simulink model "ejemplo_simulink_completo_vel_lineal_2"  (R2018a)
settings: Solver=FixedStepDiscrete  StartTime=0.0  StopTime=inf  FixedStep=0.001  RelTol=1e-3  EnableMultiTasking=on
libraries: vrlib x1, aerolibanimutils x1
settings Model: Creator=PC  LastModifiedBy=emder
settings OptimizationCC: LifeSpan=inf
settings DebuggingCC: SFUnexpectedBacktrackingDiag=warning  SFNoUnconditionalDefaultTransitionDiag=warning  SFExecutionAtInitializationDiag=none
settings CodeAppCC: StateflowObjectComments=on
settings GRTTargetCC: TargetLangStandard=C89/C90 (ANSI)  GeneratePreprocessorConditionals=Disable all
settings ConfigComp: CovMetricSettings=dw  CovHtmlReporting=on  CovSaveCumulativeToWorkspaceVar=on  CovSaveSingleToWorkspaceVar=on  CovExternalEMLEnable=off

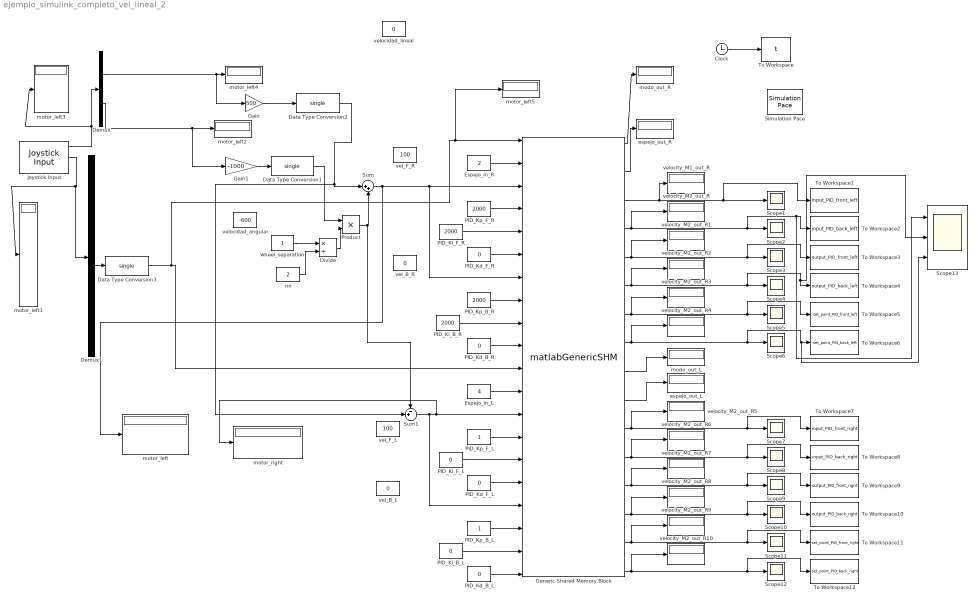
== system ejemplo_simulink_completo_vel_lineal_2 ==
  Clock : Clock
  Data Type Conversion1 : DataTypeConversion  OutDataTypeStr=single
  Data Type Conversion2 : DataTypeConversion  OutDataTypeStr=single
  Data Type Conversion3 : DataTypeConversion  OutDataTypeStr=single
  Demux : Demux  Outputs=5
  Demux1 : Demux  Outputs=10
  Divide : Product  Inputs=*/
  Espejo_in_L : Constant  Value=4  OutDataTypeStr=single
  Espejo_in_R : Constant  Value=2  OutDataTypeStr=single
  Gain : Gain  Gain=500
  Gain1 : Gain  Gain=-1000
  Generic Shared Memory Block : S-Function  FunctionName=matlabGenericSHM  Parameters=nombre,dispositivo,vecE,vecS,tipoE,tipoS,ts  SFunctionDeploymentMode=off  EnableBusSupport=off  mask(Generic Share Memory block V2.0){nombre='ARDUINO', dispositivo=1, vecE=[1 1 1 1 1 1 1 1 1 1 1 1 1 1 1 1 1 1 1 1], vecS=[1 1 1 1 1 1 1 1 1 1 1 1 1 1 1 1], tipoE=['f' 'f' 'f' 'f' 'f' 'f' 'f' 'f' 'f' 'f' 'f' 'f' 'f' 'f' 'f' 'f' 'f' 'f' 'f' 'f'], tipoS=['f' 'f' 'f' 'f' 'f' 'f' 'f' 'f' 'f' 'f' 'f' 'f' 'f' 'f' 'f' 'f'], ts=-1}
      mask prompts: nombre "Share Memory base name"; dispositivo "Device Number"; vecE "Sizes input vector"; vecS "Sizes output vector"; tipoE "Data Types Inputs"; tipoS "Data Types Outputs"; ts "Sample Time"
      mask help:
      | This block allows Simulink communication with external processes through shared memory. It works on Unix and Windows.
      | More information in Help.
      mask Help:
      | Share Memory base name (nombre): It's the base string of share memory ej 'robot'
      | Device Number (dispositivo): integer that identifies the device between multiple in use
      | Two shared memorys are created with names:
      | "%name_entrada_%dispositivo" for the device input (writing)
      | "%name_salida_%dispositivo" for the device output (reading)
      | Sizes input vector (vecE)  : array that specify the number of inputs (array dimension) and the inputs size (array values)
      | Sizes output vector  (vecS): array that specify the number of outputs (array dimension) and the outputs size (array values)
      | Data types input(tipoE): char array that specify each input types
      | Data types output (tipoS): char array that specify each output types
      | Allowed types are:
      | ('f'=float, 'd'=double, 'i'=int32, 'c'=char, 'C'= unsigned char, 'I'=unsigned int)
      | Example.
      | Suppose the following parameters:
      | nombre='exampleMemory'
      | dispositivo=10
      | vecE=[3 2 1]
      | vecS=[6 5 7 8]
      | tipoE=['f' 'I' 'c']
      | tipoS=['C' 'i' 'd' 'd']
      | 
      | Two Share Memories are created with names:
      | "exampleMemory_entrada_10" (block input)
      | "exampleMemory_salida_10"  (block output)
      | 3 inputs are created:
      |  1° Dimension 3, type "unsigned char"
      |  2° Dimension 2, type "int"
      |  3° Dimension 1, type "char"
      | 4 outputs are created:
      |  1° Dimension 6, type "float"
      |  2° Dimension 5, type "unsigned int"
      |  3° Dimension 7, type "double"
      |  3° Dimension 8, type "double"
      mask Display: image('shmem.jpg')
  Joystick Input : vrlib/Joystick Input  joyid=1  adjustports=on  forcefeed=off
      settings: SourceProductBaseCode=VR
  PID_Kd_B_L : Constant  Value=0  OutDataTypeStr=single
  PID_Kd_B_R : Constant  Value=0  OutDataTypeStr=single
  PID_Kd_F_L : Constant  Value=0  OutDataTypeStr=single
  PID_Kd_F_R : Constant  Value=0  OutDataTypeStr=single
  PID_Ki_B_L : Constant  Value=0  OutDataTypeStr=single
  PID_Ki_B_R : Constant  Value=2000  OutDataTypeStr=single
  PID_Ki_F_L : Constant  Value=0  OutDataTypeStr=single
  PID_Ki_F_R : Constant  Value=2000  OutDataTypeStr=single
  PID_Kp_B_L : Constant  OutDataTypeStr=single
  PID_Kp_B_R : Constant  Value=2000  OutDataTypeStr=single
  PID_Kp_F_L : Constant  OutDataTypeStr=single
  PID_Kp_F_R : Constant  Value=2000  OutDataTypeStr=single
  Product : Product
  Scope{1..12} (12 alike) : Scope
  Scope13 : Scope  NumInputPorts=3
  Simulation Pace : aerolibanimutils/Simulation Pace  SimulationPace=1  SleepMode=MATLAB Thread  OutputPaceError=off  SampleTime=-1
  Sum : Sum  Inputs=|++
  Sum1 : Sum  Inputs=-+|
  To Workspace : ToWorkspace  VariableName=t  SampleTime=-1
      settings: Save2DSignal=2-D array (concatenate along first dimension)
  To Workspace1 : ToWorkspace  VariableName=input_PID_front_left  SampleTime=-1
      settings: Save2DSignal=2-D array (concatenate along first dimension)
  To Workspace10 : ToWorkspace  VariableName=output_PID_back_right  SampleTime=-1
      settings: Save2DSignal=2-D array (concatenate along first dimension)
  To Workspace11 : ToWorkspace  VariableName=set_point_PID_front_right  SampleTime=-1
      settings: Save2DSignal=2-D array (concatenate along first dimension)
  To Workspace12 : ToWorkspace  VariableName=set_point_PID_back_right  SampleTime=-1
      settings: Save2DSignal=2-D array (concatenate along first dimension)
  To Workspace2 : ToWorkspace  VariableName=input_PID_back_left  SampleTime=-1
      settings: Save2DSignal=2-D array (concatenate along first dimension)
  To Workspace3 : ToWorkspace  VariableName=output_PID_front_left  SampleTime=-1
      settings: Save2DSignal=2-D array (concatenate along first dimension)
  To Workspace4 : ToWorkspace  VariableName=output_PID_back_left  SampleTime=-1
      settings: Save2DSignal=2-D array (concatenate along first dimension)
  To Workspace5 : ToWorkspace  VariableName=set_point_PID_front_left  SampleTime=-1
      settings: Save2DSignal=2-D array (concatenate along first dimension)
  To Workspace6 : ToWorkspace  VariableName=set_point_PID_back_left  SampleTime=-1
      settings: Save2DSignal=2-D array (concatenate along first dimension)
  To Workspace7 : ToWorkspace  VariableName=input_PID_front_right  SampleTime=-1
      settings: Save2DSignal=2-D array (concatenate along first dimension)
  To Workspace8 : ToWorkspace  VariableName=input_PID_back_right  SampleTime=-1
      settings: Save2DSignal=2-D array (concatenate along first dimension)
  To Workspace9 : ToWorkspace  VariableName=output_PID_front_right  SampleTime=-1
      settings: Save2DSignal=2-D array (concatenate along first dimension)
  espejo_out_L : Display
  espejo_out_R : Display
  modo_out_L : Display
  modo_out_R : Display
  motor_left{,1..5} (6 alike) : Display
  motor_right : Display
  nn : Constant  Value=2  OutDataTypeStr=single
  vel_B_L : Constant  Value=0  OutDataTypeStr=single
  vel_B_R : Constant  Value=0  OutDataTypeStr=single
  vel_F_L : Constant  Value=100  OutDataTypeStr=single
  vel_F_R : Constant  Value=100  OutDataTypeStr=single
  velocidad_angular : Constant  Value=-600  OutDataTypeStr=single
  velocidad_lineal : Constant  Value=0  OutDataTypeStr=single
  "velocity_M1_out_R " : Display
      settings: Decimation=3
  velocity_M2_out_R{,1..10} (11 alike) : Display
  wheel_separation : Constant  OutDataTypeStr=single
  wires:
  Generic Shared Memory Block/1 -> modo_out_R/1
  Generic Shared Memory Block/2 -> espejo_out_R/1
  Espejo_in_R/1 -> Generic Shared Memory Block/2
  Generic Shared Memory Block/3 -> To Workspace1/1, Scope1/1, "velocity_M1_out_R "/1
  Generic Shared Memory Block/4 -> Scope2/1, Scope13/1, To Workspace2/1, velocity_M2_out_R/1
  Divide/1 -> Product/2
  wheel_separation/1 -> Divide/1
  nn/1 -> Divide/2
  Product/1 -> Sum1/1, Sum/2
  Sum/1 -> motor_left/1, Generic Shared Memory Block/3, Generic Shared Memory Block/7
  PID_Kp_F_R/1 -> Generic Shared Memory Block/4
  PID_Ki_F_R/1 -> Generic Shared Memory Block/5
  PID_Kd_F_R/1 -> Generic Shared Memory Block/6
  PID_Kp_B_R/1 -> Generic Shared Memory Block/8
  PID_Ki_B_R/1 -> Generic Shared Memory Block/9
  PID_Kd_B_R/1 -> Generic Shared Memory Block/10
  PID_Ki_B_L/1 -> Generic Shared Memory Block/19
  PID_Kd_B_L/1 -> Generic Shared Memory Block/20
  PID_Kp_B_L/1 -> Generic Shared Memory Block/18
  Espejo_in_L/1 -> Generic Shared Memory Block/12
  Sum1/1 -> motor_right/1, Generic Shared Memory Block/13, Generic Shared Memory Block/17
  PID_Kp_F_L/1 -> Generic Shared Memory Block/14
  PID_Ki_F_L/1 -> Generic Shared Memory Block/15
  PID_Kd_F_L/1 -> Generic Shared Memory Block/16
  Joystick Input/1 -> motor_left3/1, Demux/1
  Demux/4 -> Gain1/1, motor_left2/1
  Joystick Input/2 -> Demux1/1, motor_left1/1
  Demux/2 -> Gain/1, motor_left4/1
  Gain/1 -> Data Type Conversion2/1
  Gain1/1 -> Data Type Conversion1/1
  Data Type Conversion1/1 -> Product/1
  Data Type Conversion2/1 -> Sum1/2, Sum/1
  Demux1/6 -> Data Type Conversion3/1
  Data Type Conversion3/1 -> motor_left5/1, Generic Shared Memory Block/1, Generic Shared Memory Block/11
  Clock/1 -> To Workspace/1
  Generic Shared Memory Block/5 -> Scope3/1, To Workspace3/1, velocity_M2_out_R1/1
  Generic Shared Memory Block/6 -> Scope4/1, Scope13/2, To Workspace4/1, velocity_M2_out_R2/1
  Generic Shared Memory Block/7 -> Scope5/1, To Workspace5/1, velocity_M2_out_R3/1
  Generic Shared Memory Block/8 -> Scope6/1, Scope13/3, To Workspace6/1, velocity_M2_out_R4/1
  Generic Shared Memory Block/11 -> Scope7/1, To Workspace7/1, velocity_M2_out_R5/1
  Generic Shared Memory Block/12 -> Scope8/1, To Workspace8/1, velocity_M2_out_R6/1
  Generic Shared Memory Block/13 -> Scope9/1, To Workspace9/1, velocity_M2_out_R7/1
  Generic Shared Memory Block/14 -> Scope10/1, To Workspace10/1, velocity_M2_out_R8/1
  Generic Shared Memory Block/15 -> Scope11/1, To Workspace11/1, velocity_M2_out_R9/1
  Generic Shared Memory Block/16 -> Scope12/1, To Workspace12/1, velocity_M2_out_R10/1
  Generic Shared Memory Block/9 -> modo_out_L/1
  Generic Shared Memory Block/10 -> espejo_out_L/1
